simulink model "obstacle"  (R2019b)
settings: Solver=FixedStepAuto  StartTime=0.0  StopTime=10.0  RelTol=1e-3  EnableMultiTasking=on
libraries: legoev3lib x3
settings Model: ExtModeTrigDuration=2  Creator=alumnopr18  LastModifiedBy=alumnopr18
settings SolverCC: PositivePriorityOrder=on
settings OptimizationCC: EnhancedBackFolding=on  PassReuseOutputArgsAs=Individual arguments  ZeroExternalMemoryAtStartup=off  ZeroInternalMemoryAtStartup=off  MaxStackSize=64  OptimizeBlockOrder=speed  DifferentSizesBufferReuse=on  OptimizationCustomize=off  EfficientTunableParamExpr=on
settings DebuggingCC: ParameterTunabilityLossMsg=error
settings HardwareCC: ProdBitPerPointer=32  ProdBitPerSizeT=32  ProdBitPerPtrDiffT=32  ProdLargestAtomicInteger=Long  ProdWordSize=32  ProdHWDeviceType=ARM Compatible->ARM 9
settings SFSimCC: MATLABDynamicMemAlloc=off
settings RTWCC: SystemTargetFile=ert.tlc  HardwareBoard=LEGO MINDSTORMS EV3  TLCOptions="-aInlineSetEventsForThisBaseRateFcn=TLC_FALSE -aSuppressMultiTaskScheduler=TLC_FALSE  -aRateBasedStepFcn=0"  TemplateMakefile=ert_default_tmf  GenerateReport=on  Toolchain=Sourcery G++ Lite v2009q3  IncludeHyperlinkInReport=on  LaunchReport=on  GenerateTraceInfo=on  GenerateTraceReport=on  GenerateTraceReportSl=on  GenerateTraceReportSf=on  GenerateTraceReportEml=on
settings CodeAppCC: ForceParamTrailComments=on  IgnoreCustomStorageClasses=off  OperatorAnnotations=on  SimulinkDataObjDesc=on  SFDataObjDesc=on  InsertBlockDesc=on
settings ERTTargetCC: SupportContinuousTime=on  SupportVariableSizeSignals=on

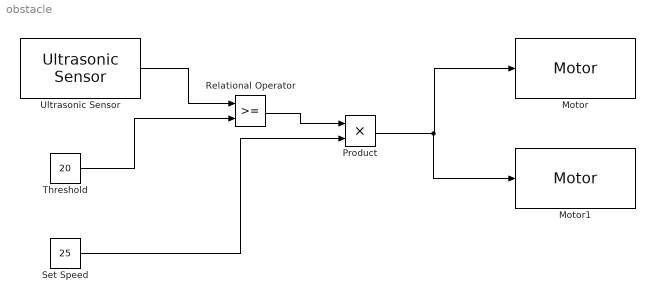
== system obstacle ==
  Motor : legoev3lib/Motor  sportNumber=B  sstopAction=Brake
  Motor1 : legoev3lib/Motor  sportNumber=C  sstopAction=Brake
  Product : Product
  Relational Operator : RelationalOperator  OutDataTypeStr=boolean  RndMeth=Simplest
  "Set Speed " : Constant  Value=25
  Threshold : Constant  Value=20
  Ultrasonic Sensor : legoev3lib/Ultrasonic Sensor  PortNumber=1  sampleTime=0.1
      settings: SourceProductName=Simulink Support Package for LEGO MINDSTORMS EV3 Hardware  SourceProductBaseCode=LEGOEV3
  wires:
  Ultrasonic Sensor/1 -> Relational Operator/1
  Threshold/1 -> Relational Operator/2
  Relational Operator/1 -> Product/1
  "Set Speed "/1 -> Product/2
  Product/1 -> Motor1/1, Motor/1
